simulink model "models1bad"  (R2022a)
settings: Solver=ode3  StartTime=0.0  StopTime=1.5  FixedStep=2e-5  MaxStep=1e-4  RelTol=1e-3
undefined symbols (not defined in the file or in its folder): J, K_1, K_2, K_3, K_4, K_i, K_u, Lm, Lr, Ls, Ml, U_dc, w0_, zp
libraries: ee_lib x11, nesl_utility x11, fl_lib x7, simulink x3
settings Model: Creator=sdani  LastModifiedBy=Family
settings SolverCC: AlgebraicLoopSolver=TrustRegion
settings DebuggingCC: SFMachineParentedDataDiag=warning
settings ModelReferenceCC: EnableRefExpFcnMdlSchedulingChecks=off
settings RTWCC: Description=Generic Real-Time Target

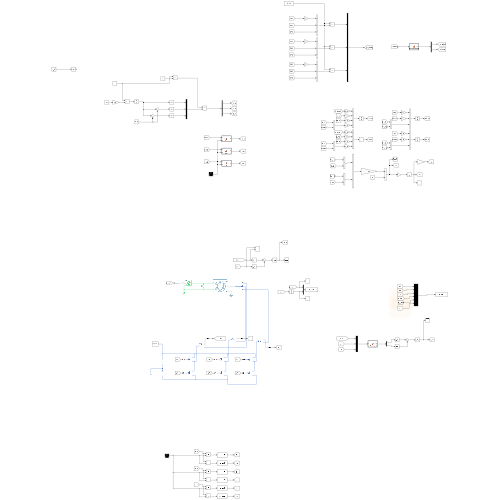
[thumbnail: Simulink's stored preview of the top-level diagram]
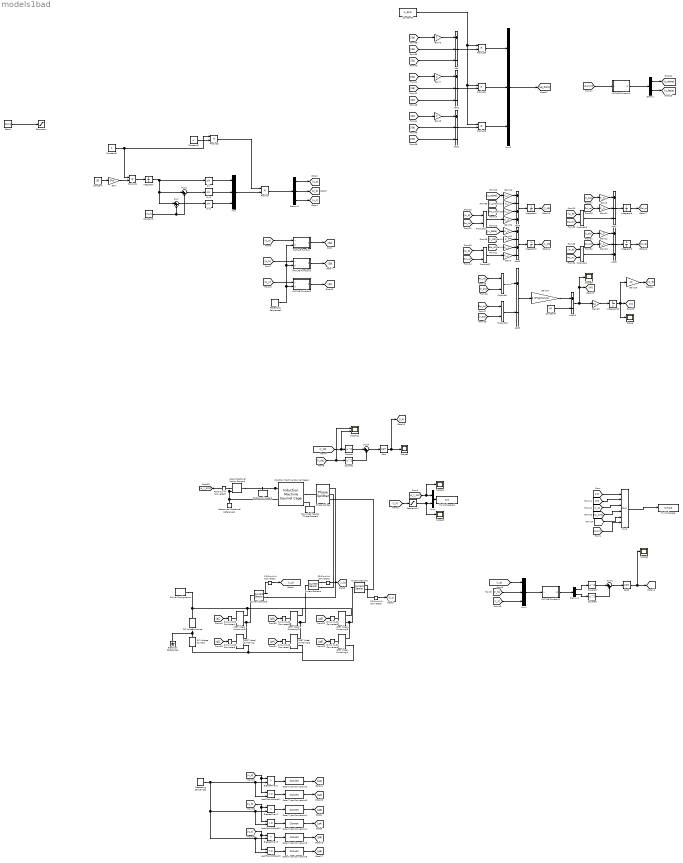
== system models1bad ==
  Add{,1..2,7} (4 alike) : Sum  Inputs=+--
  Add10 : Sum  Inputs=+-
  Add5 : Sum  Inputs=+-++
  Add6 : Sum  Inputs=+-+-
  Add8 : Sum  Inputs=+-+
  Add9 : Sum  Inputs=+-
  Constant : Constant  Value=50
  Constant1 : Constant  Value=2*pi/3
  Constant2 : Constant  Value=u
  Constant4 : Constant  Value=Ml
  Constant5 : Constant  Value=U_dc/3
  Constant6 : Constant
  Current Sensor3 : fl_lib/Electrical/Electrical Sensors/Current Sensor
      settings: SourceProductBaseCode=PW,SS,VE
  Current Sensor4 : fl_lib/Electrical/Electrical Sensors/Current Sensor
      settings: SourceProductBaseCode=PW,SS,VE
  Current Sensor5 : fl_lib/Electrical/Electrical Sensors/Current Sensor
      settings: SourceProductBaseCode=PW,SS,VE
  DC Voltage Source : ee_lib/Additional Components/SPICE Sources/DC Voltage Source  DC=U_dc*0.575 V
  DC Voltage Source1 : ee_lib/Additional Components/SPICE Sources/DC Voltage Source  DC=U_dc*0.575 V
  Data Type Conversion{1..6} (6 alike) : DataTypeConversion  SaturateOnIntegerOverflow=off  RndMeth=Floor
  Demux : Demux  Outputs=2
  Demux1 : Demux  Outputs=3
  Demux2 : Demux  Outputs=2
  Electrical Reference1 : fl_lib/Electrical/Electrical Elements/Electrical Reference
      settings: SourceProductBaseCode=PW,SS,VE
  Gain : Gain  Gain=2*pi
  Gain2 : Gain  Gain=K_i
  Gain21 : Gain  Gain=K_4
  Gain22 : Gain  Gain=K_3
  Gain23 : Gain  Gain=K_4
  Gain24 : Gain  Gain=1.5*zp*Lm/Lr
  Gain25 : Gain  Gain=1/J
  Gain26 : Gain  Gain=K_u
  Gain27 : Gain  Gain=K_i
  Gain28 : Gain  Gain=K_1
  Gain29 : Gain  Gain=zp
  Gain3 : Gain  Gain=K_1
  Gain30 : Gain  Gain=K_2
  Gain31 : Gain  Gain=K_u
  Gain4 : Gain  Gain=K_2
  Gain5 : Gain  Gain=K_3
  Gain6 : Gain  Gain=2
  Gain7 : Gain  Gain=2
  Gain8 : Gain  Gain=2
  GreaterThan1 : RelationalOperator  Operator=>  OutDataTypeStr=boolean  RndMeth=Simplest  InputSameDT=off
  GreaterThan2 : RelationalOperator  Operator=>  OutDataTypeStr=boolean  RndMeth=Simplest  InputSameDT=off
  GreaterThan3 : RelationalOperator  Operator=>  OutDataTypeStr=boolean  RndMeth=Simplest  InputSameDT=off
  Grounded Neutral (Three-Phase)1 : ee_lib/Connectors & References/Grounded Neutral (Three-Phase)
      settings: SourceProductBaseCode=PS
  IGBT (Ideal, Switching){,1..4,6} (6 alike) : ee_lib/Semiconductors & Converters/IGBT (Ideal, Switching)  Vf=0.8 V  Ron=0.001 Ohm  Goff=1e-5 1/Ohm  Vth=.5 V  diode_param=ee.enum.converters.protectiondiode.none  diode_Vf=0.8 V  diode_Ron=0.001 Ohm  diode_Goff=1e-5 1/Ohm  diode_C=50e-9 F  diode_iRM=-235 A  diode_iF=300 A  diode_idot=-50 A/us  diode_trr_param=ee.enum.converters.diodeReverseParam.trr_factor  diode_trr_factor=3  diode_trr=15 us  diode_Qrr=1500 s*uA  thermal_loss_option=ee.enum.converters.thermalLossOption.constantvalues  Von_data=[0, .1, .6, .8, 1, 1.3, 1.6, 2, 2.4; 0, .1, .7, 1, 1.2, 1.5, 1.9, 2.4, 2.8] V  Tj=[298.15, 398.15] K  Iout_data=[0, .1, 1, 5, 10, 20, 40, 70, 100] A  Eon_data=[0, .0024, .024, .12, .2, .48, 1.04, 2.16, 3.24; 0, .003, .03, .15, .25, .6, 1.3, 2.7, 4.05] * 1e-3 J  Eoff_data=[0, .0007, .0066, .033, .066, .17, .33, .83, 1.5; 0, .001, .01, .05, .1, .25, .5, 1.2, 2.2] * 1e-3 J  Tj_loss=[298.15, 398.15] K  Iout_data_loss=[0, .1, 1, 5, 10, 20, 40, 70, 100] A  Eon_scalar=22.86e-3 J  Eoff_scalar=17.14e-3 J  Voff=300 V  Iout_scalar=600 A  diodeModelType=ee.enum.converters.diodeModelType.pwl  diodeTableType=ee.enum.diode.tableType.IfMat  diode_IfMat=[.07, .12, .19, 1.75, 4.24, 7.32, 11.2; .16, .3, .72, 2.14, 4.02, 6.35, 9.12] A  diode_VfMat=[.9, 1.15, 1.25, 1.5, 1.75, 2.17, 2.6, 2.85; .58, .68, .75, 1.1, 1.38, 1.77, 2.27, 2.7] V  diode_TjVec=[25, 125] degC  diode_VfVec=[.5, .7, .9, 1.3, 1.7, 2.1, 2.5] V  diode_IfVec=[.1, .2, .5, 1, 2, 4, 7, 10] A  diode_Vr=-600 V  diode_Ls=150 nH  diode_Erec=0.03 J  thermal_network_parameterization=ee.enum.thermalNetworkTopology.external  Rth=[.08, .5] K/W  Rth_Cauer=[.08, .1, .5] K/W  Rth_Foster=[.08, .14, .22, .16] K/W  thermal_mass_parameterization=ee.enum.thermalNetwork.timeconstant  thermal_mass=[.01, .5] J/K  thermal_mass_Cauer=[.01, .1, .5] J/K  thermal_mass_Foster=[.001, .005, .05, .5] J/K  thermal_time_constant=[.001, .2] s  thermal_time_constant_Cauer=[.001, .1, .2] s  thermal_time_constant_Foster=[7e-05, .0007, .01, .08] s  thermal_mass_initial_temperatures=[25, 25] degC  thermal_mass_initial_temperatures_Cauer=[25, 25, 25] degC  junction_thermal_mass=0.01 J/K  steadyState_Foster=simscape.enum.onoff.on  Tvec_initial_Foster=[25, 25, 25, 25] degC  no_thermal_network=0  junction_temperature_specify=off  junction_temperature_priority=None  junction_temperature=25 degC  junction_temperature_nominal_specify=off  junction_temperature_nominal_unit=degC  junction_temperature_nominal_value=1  vT_specify=off  vT_priority=None  vT=0 V  vT_nominal_specify=off  vT_nominal_unit=V  vT_nominal_value=1  Qj_specify=off  Qj_priority=None  Qj=0 W  Qj_nominal_specify=off  Qj_nominal_unit=W  Qj_nominal_value=1
  Ideal Rotational Motion Sensor1 : fl_lib/Mechanical/Mechanical Sensors/Ideal Rotational Motion Sensor  wrap_angle=simscape.enum.onoff.off  offset=0 rad
      settings: SourceProductBaseCode=PW,SS,VE
  Induction Machine Squirrel Cage1 : ee_lib/Electromechanical/Asynchronous/Induction Machine Squirrel Cage  port_option=ee.enum.threePhasePort.composite  SRated=0.75 kW  VRated=220 V  FRated=50 Hz  nPolePairs=3  param_unit=ee.enum.unit.si  squirrel_cage=ee.enum.squirrelcage.Single  zero_sequence=ee.enum.park.zerosequence.exclude  initialization_option=ee.enum.asm.initialization.fluxvariables  Rs=Rs Ohm  Xls=Ls*w0_ Ohm  pu_Rs=0.0258  pu_Lls=0.0413  Rrd=Rr Ohm  Xlrd=Lr*w0_ Ohm  pu_Rrd=0.0145  pu_Llrd=0.0424  Rrd1=0.28 Ohm  Xlrd1=0.82 Ohm  Rrd2=0.28 Ohm  Xlrd2=0.82 Ohm  pu_Rrd1=0.0290  pu_Llrd1=0.0848  pu_Rrd2=0.0290  pu_Llrd2=0.0848  Xm=Lm*w0_ Ohm  pu_Lm=1.7562  X0=0.4 Ohm  pu_L0=0.0413  saturation_option=ee.enum.saturation.exclude  saturation_i=[0, 4, 9, 18, 25, 34, 50, 68, 95, 120] A  saturation_v=[0, 88, 154, 198, 220, 242, 264, 286, 308, 327] V  pu_saturation_i=[0, .176, .396, .792, 1.1, 1.496, 2.2, 2.992, 4.18, 5.28]  pu_saturation_v=[0, .4, .7, .9, 1, 1.1, 1.2, 1.3, 1.4, 1.4864]  connection_option=ee.enum.Connection.delta  angular_position_specify=off  angular_position_priority=None  angular_position=0 deg  angular_position_nominal_specify=off  angular_position_nominal_unit=deg  angular_position_nominal_value=1  pu_psids_specify=off  pu_psids_priority=None  pu_psids=0  pu_psids_nominal_specify=off  pu_psids_nominal_unit=1  pu_psids_nominal_value=1  pu_psiqs_specify=off  pu_psiqs_priority=None  pu_psiqs=0  pu_psiqs_nominal_specify=off  pu_psiqs_nominal_unit=1  pu_psiqs_nominal_value=1  pu_psi0s_specify=off  pu_psi0s_priority=None  pu_psi0s=0  pu_psi0s_nominal_specify=off  pu_psi0s_nominal_unit=1  pu_psi0s_nominal_value=1  pu_psidr_specify=off  pu_psidr_priority=None  pu_psidr=0  pu_psidr_nominal_specify=off  pu_psidr_nominal_unit=1  pu_psidr_nominal_value=1  pu_psiqr_specify=off  pu_psiqr_priority=None  pu_psiqr=0  pu_psiqr_nominal_specify=off  pu_psiqr_nominal_unit=1  pu_psiqr_nominal_value=1  pu_psidr1_specify=off  pu_psidr1_priority=None  pu_psidr1=0  pu_psidr1_nominal_specify=off  pu_psidr1_nominal_unit=1  pu_psidr1_nominal_value=1  pu_psiqr1_specify=off  pu_psiqr1_priority=None  pu_psiqr1=0  pu_psiqr1_nominal_specify=off  pu_psiqr1_nominal_unit=1  pu_psiqr1_nominal_value=1  pu_psidr2_specify=off  pu_psidr2_priority=None  pu_psidr2=0  pu_psidr2_nominal_specify=off  pu_psidr2_nominal_unit=1  pu_psidr2_nominal_value=1  pu_psiqr2_specify=off  pu_psiqr2_priority=None  pu_psiqr2=0  pu_psiqr2_nominal_specify=off  pu_psiqr2_nominal_unit=1  pu_psiqr2_nominal_value=1  psids_specify=off  psids_priority=None  psids=0 Wb  psids_nominal_specify=off  psids_nominal_unit=Wb  psids_nominal_value=1  psiqs_specify=off  psiqs_priority=None  psiqs=0 Wb  psiqs_nominal_specify=off  psiqs_nominal_unit=Wb  psiqs_nominal_value=1  psi0s_specify=off  psi0s_priority=None  psi0s=0 Wb  psi0s_nominal_specify=off  psi0s_nominal_unit=Wb  psi0s_nominal_value=1  psidr_specify=off  psidr_priority=None  psidr=0 Wb  psidr_nominal_specify=off  psidr_nominal_unit=Wb  psidr_nominal_value=1  psiqr_specify=off  psiqr_priority=None  psiqr=0 Wb  psiqr_nominal_specify=off  psiqr_nominal_unit=Wb  psiqr_nominal_value=1  psidr1_specify=off  psidr1_priority=None  psidr1=0 Wb  psidr1_nominal_specify=off  psidr1_nominal_unit=Wb  psidr1_nominal_value=1  psiqr1_specify=off  psiqr1_priority=None  psiqr1=0 Wb  psiqr1_nominal_specify=off  psiqr1_nominal_unit=Wb  psiqr1_nominal_value=1  psidr2_specify=off  psidr2_priority=None  psidr2=0 Wb  psidr2_nominal_specify=off  psidr2_nominal_unit=Wb  psidr2_nominal_value=1  psiqr2_specify=off  psiqr2_priority=None  psiqr2=0 Wb  psiqr2_nominal_specify=off  psiqr2_nominal_unit=Wb  psiqr2_nominal_value=1  slip_specify=off  slip_priority=None  slip=0  slip_nominal_specify=off  slip_nominal_unit=1  slip_nominal_value=1  real_power_generated_specify=off  real_power_generated_priority=None  real_power_generated=0 W  real_power_generated_nominal_specify=off  real_power_generated_nominal_unit=W  real_power_generated_nominal_value=1  mechanical_power_consumed_specify=off  mechanical_power_consumed_priority=None  mechanical_power_consumed=0 W  mechanical_power_consumed_nominal_specify=off  mechanical_power_consumed_nominal_unit=W  mechanical_power_consumed_nominal_value=1  Tmeas=298.15 K  alpha=3.93e-3 1/K  alpha_cage=4.4e-3 1/K  stator_thermal_mass=100 J/K  rotor_thermal_mass=200 J/K  temperatureA_specify=off  temperatureA_priority=High  temperatureA=25 degC  temperatureA_nominal_specify=off  temperatureA_nominal_unit=degC  temperatureA_nominal_value=1  temperatureB_specify=off  temperatureB_priority=High  temperatureB=25 degC  temperatureB_nominal_specify=off  temperatureB_nominal_unit=degC  temperatureB_nominal_value=1  temperatureC_specify=off  temperatureC_priority=High  temperatureC=25 degC  temperatureC_nominal_specify=off  temperatureC_nominal_unit=degC  temperatureC_nominal_value=1  temperatureR_specify=off  temperatureR_priority=High  temperatureR=25 degC  temperatureR_nominal_specify=off  temperatureR_nominal_unit=degC  temperatureR_nominal_value=1
      settings: SourceProductBaseCode=PS  InternalSimscapePortConfiguration="{\"Bottom\":[],\"Left\":[{\"id\":\"R\",\"label\":\"R\",\"type\":\"foundation.mechanical.rotational.rotational\"},{\"id\":\"C\",\"label\":\"C\",\"type\":\"foundation.mechanical.rotational.rotational\"}],\"Right\":[{\"id\":\"pu_output\",\"label\":\"pu\",\"type\":\"output\"},{\"id\":\"N1\",\"label\":\"~1\",\"type\":\"foundation.electrical.three_phase\"},{\"id\":\"N2\",\"label\":\"~2\",\"type\":\"foundation.electrical.three_phase\"}],\"Top\":[]}"
  Integrator{,1..2,8..10} (6 alike) : Integrator
  LessThanOrEqual1 : RelationalOperator  Operator=<=  OutDataTypeStr=boolean  RndMeth=Simplest  InputSameDT=off
  LessThanOrEqual2 : RelationalOperator  Operator=<=  OutDataTypeStr=boolean  RndMeth=Simplest  InputSameDT=off
  LessThanOrEqual3 : RelationalOperator  Operator=<=  OutDataTypeStr=boolean  RndMeth=Simplest  InputSameDT=off
  MATLAB Function : MATLAB Function  TreatAsAtomicUnit=on
  MATLAB Function1 : MATLAB Function  TreatAsAtomicUnit=on  SystemSampleTime=2e-5
  MATLAB Function2 : MATLAB Function  TreatAsAtomicUnit=on
  MATLAB Function3 : MATLAB Function  TreatAsAtomicUnit=on
  MATLAB Function4 : MATLAB Function  TreatAsAtomicUnit=on  SystemSampleTime=2e-5
  Mechanical Rotational Reference2 : fl_lib/Mechanical/Rotational Elements/Mechanical Rotational Reference
      settings: SourceProductBaseCode=PW,SS,VE
  Mux : Mux  Inputs=3
  Mux1 : Mux  Inputs=3
  Mux2 : Mux  Inputs=6
  Mux3 : Mux  Inputs=3
  Mux4 : Mux  Inputs=2
  PS-Simulink Converter{1..3,5} (4 alike) : nesl_utility/PS-Simulink Converter  PhysicalDomain=network_engine_domain  SubClassName=ps_output  LeftPortType=input  RightPortType=output  PseudoPeriodic=off  Frequencies=[]  VectorFormat=inherit  Unit=inherit  AffineConversion=off
      settings: SourceProductBaseCode=SS,PW,VE
  Phase Splitter : ee_lib/Connectors & References/Phase Splitter
      settings: SourceProductBaseCode=PS
  Product{,1..5,9..14} (12 alike) : Product
  Ramp : simulink/Sources/Ramp  slope=1  start=0  InitialOutput=0
  Repeating Sequence1 : simulink/Sources/Repeating Sequence  rep_seq_t=[0 1/10000 1/5000]  rep_seq_y=[-1 1 -1]
  Repeating Sequence2 : simulink/Sources/Repeating Sequence  rep_seq_t=[0 1/10000 1/5000]  rep_seq_y=[-1 1 -1]
  Rotational Inerter1 : fl_lib/Mechanical/Rotational Elements/Rotational Inerter  B=J kg*m^2  w_specify=off  w_priority=High  w=0 rad/s  w_nominal_specify=off  w_nominal_unit=rad/s  w_nominal_value=1  t_specify=off  t_priority=None  t=0 N*m  t_nominal_specify=off  t_nominal_unit=N*m  t_nominal_value=1
      settings: SourceProductBaseCode=PW,SS,VE  InternalSimscapePortConfiguration="{\"Bottom\":[],\"Left\":[{\"id\":\"R\",\"label\":\"R\",\"type\":\"foundation.mechanical.rotational.rotational\"}],\"Right\":[{\"id\":\"C\",\"label\":\"C\",\"type\":\"foundation.mechanical.rotational.rotational\"}],\"Top\":[]}"
  Saturation : Saturate  UpperLimit=1  LowerLimit=0.05
  Saturation1 : Saturate  UpperLimit=5  LowerLimit=2
  Scope{,2..5,8} (6 alike) : Scope
  Scope11 : Scope  NumInputPorts=2
  Simulink-PS Converter{4..9} (6 alike) : nesl_utility/Simulink-PS Converter  PhysicalDomain=network_engine_domain  SubClassName=ps_input  LeftPortType=input  RightPortType=output  PseudoPeriodic=off  Frequencies=[]  NoiseDistribution=none  NoiseParameters=[]  Unit=1  AffineConversion=off  FilteringAndDerivatives=provide  SimscapeFilterOrder=1  InputFilterTimeConstant=0.001  UdotUserProvided=0
      settings: SourceProductBaseCode=SS,PW,VE
  Sin : Trigonometry
  Sin1 : Trigonometry
  Sin2 : Trigonometry
  Solver Configuration : nesl_utility/Solver Configuration  PhysicalDomain=network_engine_domain  SubClassName=solver  LeftPortType=input  RightPortType=generic  Tones=[]  Harmonics=[]  SimulateNoise=off  Profile=off  UseLocalSampling=off  EnableSwitchedLinearOptims=on  FrequencyDomain=off  UseCCode=off  RelTol=0.001  AbsTol=0.001  MinStep=1e-09  ToWorkspace=off  RevertToSquareIcSolve=off  NumHomotopyIterations=100  PhasorMode=off  PhasorModeNumHarmonics=1  IndexReductionMethod=DerivativeReplacement  DoDC=off  ResidualTolerance=1e-09  UseLocalSolver=on  LocalSolverChoice=NE_TRAPEZOIDAL_ADVANCER  LocalSolverSampleTime=2e-5  DoFixedCost=on  MaxNonlinIter=3  MaxModeIter=2  ComputeImpulses=off  ImpulseIterations=2  LinearAlgebra=auto  LinearAlgebraNumThread=0  EquationFormulation=NE_TIME_EF  DelaysMemoryBudget=1024  AutomaticFiltering=on  FilteringTimeConstant=0.001  PartitionStorageMethod=AS_NEEDED  PartitionMemoryBudget=1024  PartitionMethod=ROBUST
      settings: SourceProductBaseCode=SS,PW,VE
  Sqrt : Sqrt
  Sqrt2 : Sqrt
  Square{,1,5..6} (4 alike) : Math  Operator=square
  Sum : Sum  Inputs=|++
  Sum1 : Sum  Inputs=|+-
  Sum2 : Sum  Inputs=|++
  Sum4 : Sum  Inputs=|++
  To Workspace : ToWorkspace  VariableName=simout  SaveFormat=Structure With Time  SampleTime=1e-4
  To Workspace1 : ToWorkspace  VariableName=sim  SaveFormat=Timeseries  SampleTime=-1
  wires:
  Constant/1 -> Gain/1
  Constant1/1 -> Sum1/2, Sum/2
  Sum1/1 -> Sin1/1
  Sum/1 -> Sin2/1
  Mux/1 -> Product/2
  Sin/1 -> Mux/1
  Sin1/1 -> Mux/2
  Sin2/1 -> Mux/3
  Product2/1 -> Product/1
  Integrator/1 -> Sum1/1, Sum/1, Sin/1
  Product/1 -> Demux1/1
  Demux1/1 -> [u_a]
  Demux1/2 -> [u_b]
  Demux1/3 -> [u_c]
  Gain/1 -> Product1/2
  Product1/1 -> Integrator/1
  Constant2/1 -> Product2/2
  Ramp/1 -> Saturation/1
  Mux2/1 -> To Workspace/1
  [M] -> Mux2/2
  Sqrt2/1 -> Scope8/1, [i_s_sim]
  [w_sim] -> Mux2/4
  [w] -> Mux2/1
  [i_s] -> Mux2/3
  [i_s_sim] -> Mux2/5
  Square5/1 -> Sum2/1
  Sum2/1 -> Sqrt2/1
  Sum4/1 -> Sqrt/1
  [i_b] -> Mux1/2
  Square6/1 -> Sum2/2
  Demux2/1 -> Square5/1
  [i_c] -> Mux1/3
  [i_sb] -> Scope11/1, Square1/1
  Square1/1 -> Sum4/2
  [i_sa] -> Scope11/2, Square/1
  Demux2/2 -> Square6/1
  Square/1 -> Sum4/1
  [i_a] -> Mux1/1
  Mux1/1 -> MATLAB Function1/1(u)
  MATLAB Function1/1(u2) -> Demux2/1
  Sqrt/1 -> [i_s], Scope2/1
  [u_alpha] -> Gain26/1
  [Psi_rb] -> Gain23/1
  Constant4/1 -> Add10/2
  Gain25/1 -> Integrator10/1
  Product14/1 -> Add8/3
  [Psi_ra] -> Product14/2
  [w_e] -> Product13/1
  Gain21/1 -> Add7/2
  [Psi_rb] -> Product13/2
  Gain4/1 -> Add6/4
  [Psi_ra] -> Gain21/1
  Gain28/1 -> Add5/3
  [Psi_ra] -> Product12/2
  Gain30/1 -> Add5/4
  Gain5/1 -> Add7/1
  Gain31/1 -> Add6/1
  Gain23/1 -> Add8/2
  [Psi_ra] -> Product9/1
  [w_e] -> Product11/1
  Gain3/1 -> Add6/3
  [w_e] -> Product14/1
  Add8/1 -> Integrator9/1
  Gain2/1 -> Add6/2
  Product11/1 -> Gain30/1
  [Psi_ra] -> Gain28/1
  [i_sb] -> Gain2/1
  Integrator1/1 -> [i_sa]
  Product12/1 -> Gain4/1
  [Psi_rb] -> Gain3/1
  Integrator8/1 -> [Psi_ra]
  [u_beta] -> Gain31/1
  [i_sb] -> Gain22/1
  Product9/1 -> Add9/1
  Add10/1 -> Gain25/1, Scope3/1, [M]
  [i_sa] -> Gain5/1
  Gain24/1 -> Add10/1
  Integrator10/1 -> Scope/1, Gain29/1, [w]
  [Psi_rb] -> Product11/2
  Gain29/1 -> [w_e]
  Gain26/1 -> Add5/1
  Product13/1 -> Add7/3
  [i_sa] -> Gain27/1
  Add5/1 -> Integrator1/1
  Gain22/1 -> Add8/1
  [Psi_rb] -> Product10/1
  Add6/1 -> Integrator2/1
  [w_e] -> Product12/1
  Integrator9/1 -> [Psi_rb]
  Add9/1 -> Gain24/1
  [i_sb] -> Product9/2
  Add7/1 -> Integrator8/1
  [i_sa] -> Product10/2
  Product10/1 -> Add9/2
  Gain27/1 -> Add5/2
  Integrator2/1 -> [i_sb]
  [u_a] -> MATLAB Function/1(u)
  [u_b] -> MATLAB Function2/1(u)
  MATLAB Function2/1(S) -> [Sb]
  [u_c] -> MATLAB Function3/1(u)
  MATLAB Function3/1(S) -> [Sc]
  Repeating Sequence1/1 -> MATLAB Function3/2(tri), MATLAB Function2/2(tri), MATLAB Function/2(tri)
  [Sa] -> Gain6/1
  Gain6/1 -> Add/1
  [Sb] -> Add/2
  [Sc] -> Add/3
  Add/1 -> Product3/2
  Constant5/1 -> Product5/1, Product4/1, Product3/1
  [Sa] -> Add1/2
  [Sc] -> Add1/3
  [Sb] -> Gain7/1
  Add1/1 -> Product4/2
  Gain7/1 -> Add1/1
  Add2/1 -> Product5/2
  Gain8/1 -> Add2/1
  [Sb] -> Add2/3
  [Sa] -> Add2/2
  [Sc] -> Gain8/1
  Product3/1 -> Mux3/1
  Product4/1 -> Mux3/2
  Product5/1 -> Mux3/3
  Mux3/1 -> [u3_PWM]
  [u3_PWM] -> MATLAB Function4/1(u)
  MATLAB Function4/1(u2) -> Demux/1
  Demux/2 -> [u_beta]
  Demux/1 -> [u_alpha]
  Constant6/1 -> Product2/1, Product1/1
  MATLAB Function/1(S) -> [Sa]
  [g1] -> Simulink-PS Converter4/1
  [g2] -> Simulink-PS Converter5/1
  [g3] -> Simulink-PS Converter6/1
  [g4] -> Simulink-PS Converter7/1
  [g5] -> Simulink-PS Converter8/1
  [g6] -> Simulink-PS Converter9/1
  [u_a] -> LessThanOrEqual1/1, GreaterThan1/1
  GreaterThan1/1 -> Data Type Conversion2/1
  Data Type Conversion2/1 -> [g1]
  Data Type Conversion3/1 -> [g2]
  LessThanOrEqual1/1 -> Data Type Conversion3/1
  [u_b] -> LessThanOrEqual2/1, GreaterThan2/1
  Data Type Conversion4/1 -> [g4]
  LessThanOrEqual2/1 -> Data Type Conversion4/1
  GreaterThan2/1 -> Data Type Conversion1/1
  Data Type Conversion1/1 -> [g3]
  [u_c] -> LessThanOrEqual3/1, GreaterThan3/1
  Data Type Conversion6/1 -> [g6]
  LessThanOrEqual3/1 -> Data Type Conversion6/1
  Repeating Sequence2/1 -> LessThanOrEqual3/2, GreaterThan3/2, LessThanOrEqual2/2, GreaterThan2/2, LessThanOrEqual1/2, GreaterThan1/2
  GreaterThan3/1 -> Data Type Conversion5/1
  Data Type Conversion5/1 -> [g5]
  PS-Simulink Converter1/1 -> [i_a]
  PS-Simulink Converter2/1 -> [i_b]
  PS-Simulink Converter3/1 -> [i_c]
  [M_sim] -> Mux2/6
  Mux4/1 -> To Workspace1/1
  [w_r_sim] -> Scope4/1, Mux4/1
  [i_c] -> Saturation1/1
  PS-Simulink Converter5/1 -> [w_r_sim]
  Saturation1/1 -> Scope5/1, Mux4/2
  connections:
  Electrical Reference1/LConn1 -- DC Voltage Source/RConn1 -- DC Voltage Source1/LConn1
  "IGBT (Ideal, Switching)6"/LConn1 -- Simulink-PS Converter4/RConn1
  "IGBT (Ideal, Switching)"/LConn1 -- Simulink-PS Converter5/RConn1
  "IGBT (Ideal, Switching)2"/LConn1 -- Simulink-PS Converter7/RConn1
  "IGBT (Ideal, Switching)1"/LConn1 -- Simulink-PS Converter6/RConn1
  "IGBT (Ideal, Switching)4"/LConn1 -- Simulink-PS Converter9/RConn1
  "IGBT (Ideal, Switching)3"/LConn1 -- Simulink-PS Converter8/RConn1
  DC Voltage Source/LConn1 -- Solver Configuration/RConn1 -- "IGBT (Ideal, Switching)6"/RConn1 -- "IGBT (Ideal, Switching)3"/RConn1 -- "IGBT (Ideal, Switching)1"/RConn1
  Current Sensor3/LConn1 -- "IGBT (Ideal, Switching)"/RConn1 -- "IGBT (Ideal, Switching)6"/RConn2
  "IGBT (Ideal, Switching)4"/RConn2 -- "IGBT (Ideal, Switching)2"/RConn2 -- "IGBT (Ideal, Switching)"/RConn2 -- DC Voltage Source1/RConn1
  Current Sensor4/LConn1 -- "IGBT (Ideal, Switching)2"/RConn1 -- "IGBT (Ideal, Switching)1"/RConn2
  Current Sensor5/LConn1 -- "IGBT (Ideal, Switching)4"/RConn1 -- "IGBT (Ideal, Switching)3"/RConn2
  Current Sensor3/RConn2 -- Phase Splitter/RConn1
  Current Sensor4/RConn2 -- Phase Splitter/RConn2
  Current Sensor5/RConn2 -- Phase Splitter/RConn3
  Current Sensor3/RConn1 -- PS-Simulink Converter1/LConn1
  Current Sensor4/RConn1 -- PS-Simulink Converter2/LConn1
  PS-Simulink Converter3/LConn1 -- Current Sensor5/RConn1
  Induction Machine Squirrel Cage1/LConn1 -- Ideal Rotational Motion Sensor1/LConn1 -- Rotational Inerter1/LConn1
  Ideal Rotational Motion Sensor1/RConn1 -- Mechanical Rotational Reference2/LConn1 -- Rotational Inerter1/RConn1 -- Induction Machine Squirrel Cage1/LConn2
  Grounded Neutral (Three-Phase)1/LConn1 -- Induction Machine Squirrel Cage1/RConn3
  PS-Simulink Converter5/LConn1 -- Ideal Rotational Motion Sensor1/RConn2
  Induction Machine Squirrel Cage1/RConn2 -- Phase Splitter/LConn1

== matlab function models1bad/MATLAB Function ==
  data: u input; S output; tri input
function S = fcn(u, tri)
if u >= tri
    S = 1;
else
    S = 0;
end

== matlab function models1bad/MATLAB Function2 ==
  data: u input; S output; tri input
function S = fcn(u, tri)
if u >= tri
    S = 1;
else
    S = 0;
end

== matlab function models1bad/MATLAB Function3 ==
  data: u input; S output; tri input
function S = fcn(u, tri)
if u >= tri
    S = 1;
else
    S = 0;
end

== matlab function models1bad/MATLAB Function4 ==
  data: u input; u2 output
function u2 = abc2alpha_beta(u)

u2 = [2/3 -1/3 -1/3;
    0 1/sqrt(3) -1/sqrt(3)]*u;
end

== matlab function models1bad/MATLAB Function1 ==
  data: u input; u2 output
function u2 = abc2alpha_beta(u)

u2 = [2/3 -1/3 -1/3;
    0 1/sqrt(3) -1/sqrt(3)]*u;
end
